simulink model "digitalize"  (Simulink 8.2)
settings: Solver=ode45  StartTime=0.0  StopTime=10.0  RelTol=1e-3
libraries: commsrccod2 x2, dsparch4 x2
settings Model: Creator=Yi_Liu  LastModifiedBy=Yi_Liu
settings DataIOCC: SignalLoggingSaveFormat=Dataset
settings OptimizationCC: ExpressionDepthLimit=128
settings DebuggingCC: FcnCallInpInsideContextMsg=EnableAllAsError  StateNameClashWarn=none
settings GRTTargetCC: CombineOutputUpdateFcns=on  GRTInterface=off

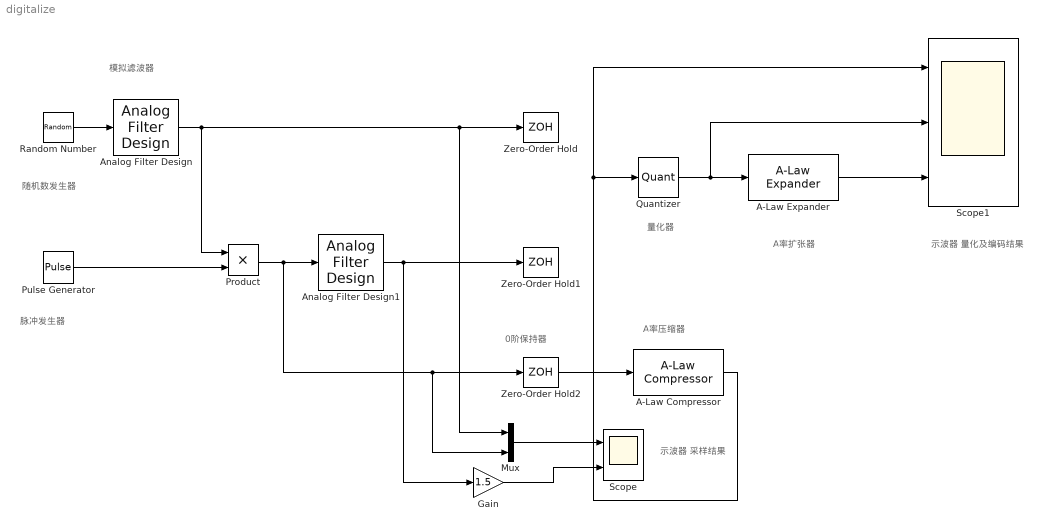
== system digitalize ==
  note: 0阶保持器
  note: A率扩张器
  note: 量化器
  note: A率压缩器
  note: 示波器
      | 量化及编码结果
  note: 示波器
      | 采样结果
  note: 脉冲发生器
  note: 模拟滤波器
  note: 随机数发生器
  A-Law Compressor : commsrccod2/A-Law Compressor  A=87.6  V=1
  A-Law Expander : commsrccod2/A-Law Expander  A=87.6  V=1
  Analog Filter Design : dsparch4/Analog Filter Design  method=Butterworth  filttype=Lowpass  N=10  Wlo=2*pi*200  Whi=80  Rp=2  Rs=40
  Analog Filter Design1 : dsparch4/Analog Filter Design  method=Butterworth  filttype=Lowpass  N=10  Wlo=2*pi*200  Whi=80  Rp=2  Rs=40
  Gain : Gain  Gain=1.5  SampleTime=0.00025
  Mux : Mux  Inputs=2
  Product : Product
  Pulse Generator : DiscretePulseGenerator  Period=10  PulseWidth=5  SampleTime=0.0001
  Quantizer : Quantizer  QuantizationInterval=0.125  LinearizeAsGain=off  SampleTime=0.1
  Random Number : RandomNumber  Seed=16  SampleTime=0.01
  Scope : Scope  NumInputPorts=2
      settings: YMin=-5~-5  YMax=5~5
  Scope1 : Scope  NumInputPorts=3
      settings: YMin=-2~-5~-5  YMax=2~5~5
  Zero-Order Hold : ZeroOrderHold  SampleTime=0.00025
  Zero-Order Hold1 : ZeroOrderHold  SampleTime=0.1
  Zero-Order Hold2 : ZeroOrderHold  SampleTime=0.1
  wires:
  Random Number/1 -> Analog Filter Design/1
  Pulse Generator/1 -> Product/2
  Analog Filter Design/1 -> Mux/1, Zero-Order Hold/1, Product/1
  Analog Filter Design1/1 -> Gain/1, Zero-Order Hold1/1
  Mux/1 -> Scope/1
  Gain/1 -> Scope/2
  Quantizer/1 -> Scope1/2, A-Law Expander/1
  Product/1 -> Analog Filter Design1/1, Mux/2, Zero-Order Hold2/1
  A-Law Compressor/1 -> Scope1/1, Quantizer/1
  A-Law Expander/1 -> Scope1/3
  Zero-Order Hold2/1 -> A-Law Compressor/1
